simulink model "btPackTest"  (R2015b)
settings: Solver=FixedStepDiscrete  StartTime=0.0  StopTime=Inf  RelTol=1e-3
libraries: freescalecupcompanionlib x1, bluetoothLibrary x1
settings Model: SimulationMode=external  ExtModeTrigDuration=5  Creator=dc315  LastModifiedBy=dc315
settings OptimizationCC: OptimizeModelRefInitCode=on  LifeSpan=1  MaxStackSize=64
settings HardwareCC: ProdBitPerPointer=32  ProdLargestAtomicInteger=Long  ProdLargestAtomicFloat=Double  ProdWordSize=32  ProdHWDeviceType=ARM Compatible->ARM Cortex
settings RTWCC: SystemTargetFile=ert.tlc  TemplateMakefile=ert_default_tmf  Description=Embedded Coder  Toolchain=GNU Tools for ARM Embedded Processors
settings CodeAppCC: IgnoreCustomStorageClasses=off

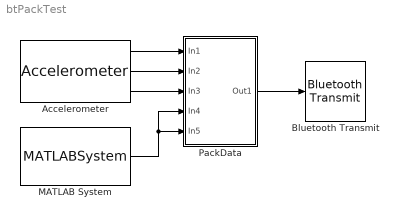
== system btPackTest ==
  Accelerometer : freescalecupcompanionlib/Accelerometer  SampleTime=0.01
  Bluetooth Transmit : bluetoothLibrary/Bluetooth Transmit  baudRate=9600
  MATLAB System : MATLABSystem  System=freedomboard.rpmSensor  SimulateUsing=Code generation
      mask Type: freedomboard.rpmSensor
      mask Display:
      | disp('rpmSensor');
      | port_label('output',1,'rpm');
  PackData : Subsystem
  wires:
  PackData/1(Out1) -> Bluetooth Transmit/1
  Accelerometer/1 -> PackData/1(In1)
  Accelerometer/2 -> PackData/2(In2)
  Accelerometer/3 -> PackData/3(In3)
  MATLAB System/1 -> PackData/5(In5), PackData/4(In4)

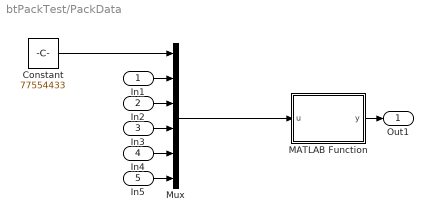
== system btPackTest/PackData ==
  In1 : Inport
  In2 : Inport  Port=2
  In3 : Inport  Port=3
  In4 : Inport  Port=4
  In5 : Inport  Port=5
  Constant : Constant  Value=77554433
  MATLAB Function : MATLAB Function  TreatAsAtomicUnit=on
  Mux : Mux  Inputs=6
  Out1 : Outport
  wires:
  Mux/1 -> MATLAB Function/1(u)
  Constant/1 -> Mux/1
  MATLAB Function/1(y) -> Out1/1
  In3/1 -> Mux/4
  In2/1 -> Mux/3
  In4/1 -> Mux/5
  In5/1 -> Mux/6
  In1/1 -> Mux/2

== matlab function btPackTest/PackData/MATLAB Function ==
  data: u input; y output
function y = fcn(u)
%#codegen

y = typecast(u,'uint8');
